simulink library "ControlLib"  (R2023a)
settings: Solver=VariableStepAuto  StartTime=0.0  StopTime=10.0  RelTol=1e-3
undefined symbols (not defined in the file): DiscIntNeverNeededParam
Description:
  | This block library contains common controllers for use by models in the project.
settings Model: Creator=The MathWorks, Inc.  LastModifiedBy=The MathWorks, Inc.
settings SolverCC: AlgebraicLoopSolver=TrustRegion
settings DataIOCC: ReturnWorkspaceOutputs=off
settings DebuggingCC: UnconnectedInputMsg=warning  UnconnectedOutputMsg=warning  UnconnectedLineMsg=warning  PregeneratedLibrarySubsystemCodeDiagnostic=none  ArithmeticOperatorsInVariantConditions=warning
settings ModelReferenceCC: EnableRefExpFcnMdlSchedulingChecks=on
settings SFSimCC: SimUseLocalCustomCode=off  CustomCodeUndefinedFunction=UseInterfaceOnly
settings RTWCC: RTWUseLocalCustomCode=off
settings CodeAppCC: StateflowObjectComments=on

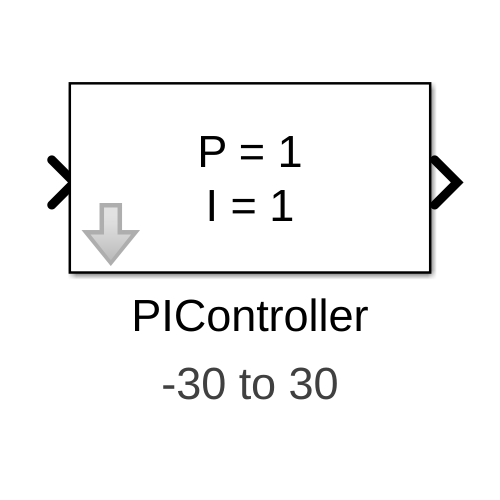
[thumbnail: Simulink's stored preview of the top-level diagram]
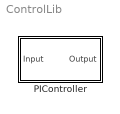
== system ControlLib ==
  PIController : Subsystem  Tag=FilterWizardSubSystem  mask(PI Controller){kp=1, ki=1, hi=30, lo=-30, ts=0.01}
      mask prompts: kp "Proportional gain"; ki "Integral gain"; hi "Upper limit"; lo "Lower limit"; ts "Sample time"
      mask help: Discrete PI controller.
      settings: AttributesFormatString=%<lo> to %<hi>  ErrorFcn=dspFilterRealizedInBasicElemsAlgLoopErrFcnCallback
      mask Display: disp(['P = ',num2str(kp),char(10),'I = ',num2str(ki)])

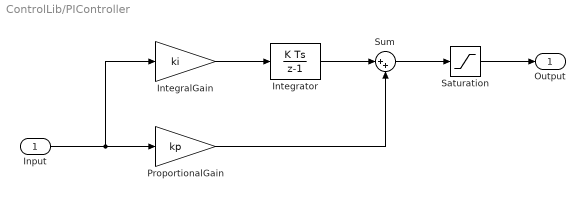
== system ControlLib/PIController ==
  Input : Inport
  IntegralGain : Gain  Gain=ki
  Integrator : DiscreteIntegrator  SampleTime=ts  LimitOutput=on  UpperSaturationLimit=hi  LowerSaturationLimit=lo  ICPrevOutput=DiscIntNeverNeededParam  ICPrevScaledInput=DiscIntNeverNeededParam
  ProportionalGain : Gain  Gain=kp
  Saturation : Saturate  UpperLimit=hi  LowerLimit=lo
  Sum : Sum  Inputs=|++
  Output : Outport  VectorParamsAs1DForOutWhenUnconnected=off
  wires:
  Sum/1 -> Saturation/1
  IntegralGain/1 -> Integrator/1
  Integrator/1 -> Sum/1
  ProportionalGain/1 -> Sum/2
  Saturation/1 -> Output/1
  Input/1 -> IntegralGain/1, ProportionalGain/1
